simulink model "vertical_smm_with_lqr_3d"  (R2015a)
settings: Solver=FixedStepDiscrete  StartTime=0.0  StopTime=inf  FixedStep=sample_time  RelTol=1e-3
values from neighbouring files (symbols this model uses):
  forward_dx_of_dxstar = [-1.33147741515 -1.28147741462 -1.23147741409 -1.18147741356 -1.13147741303 -1.0814774125 -1.03147741197 -0.981477411445 -0.931477410916 -0.881477410388 -0.831477409975 -0.781477409737 ... (28413 elements, 41x21x33)]    [ref_trajs.mat]
  forward_x_of_dxstar = [0.245075236011 0.237749717983 0.230424199955 0.223098681927 0.215773163898 0.20844764587 0.201122127842 0.193796609813 0.186471091785 0.179145573757 0.171820055745 0.164494537786 ... (28413 elements, 41x21x33)]    [ref_trajs.mat]
  target_dx_range = [-1 -0.95 -0.9 -0.85 -0.8 -0.75 -0.7 -0.65 -0.6 -0.55 -0.5 -0.45 ... (41 elements, 1x41)]    [ref_trajs.mat]
undefined symbols (not defined in the file or in its folder): A_kalman_fourbar_gear, A_kalman_transverse, A_kalman_vertical, A_lpf_dtau, A_lpf_fourbar_angles, A_lpf_imu, A_lpf_lateral_angle, A_lpf_leg_spring, B1_lpf_dtau, B1_lpf_fourbar_angles, B1_lpf_imu, B1_lpf_lateral_angle, B1_lpf_leg_spring, B2_lpf_dtau, B2_lpf_fourbar_angles, B2_lpf_imu, B2_lpf_lateral_angle, B2_lpf_leg_spring, B_dx_versus_x0, B_kalman_fourbar_gear, B_kalman_transverse, B_kalman_vertical, backwards_K_front_of_t_row1, backwards_K_front_of_t_row2, backwards_K_sag_of_t, backwards_P_front_of_t, backwards_P_sag_of_t, C_kalman_fourbar_gear, C_kalman_transverse, C_kalman_vertical, com_leg_motor, com_torso, contact_threshold, control_start_time, d_ankle_to_foot, d_vertical_com, desired_com_forward_velocity, desired_com_lateral_velocity, desired_initial_leg_roll_left, desired_initial_leg_roll_right, desired_lateral_symmetry_angle, desired_standing_torso_pitch, desired_standing_torso_roll, desired_standing_z, desired_torso_pitch, desired_torso_roll, Discrete, fcut_contact, g, HIP_MTR_MAX_CONT_TORQUE, HIP_MTR_MAX_TORQUE, i_leg_motor, i_robot, i_torso, initial_dx_estimate, initial_dy_estimate, initial_dz_estimate, initial_z_estimate, j_motor, K_left_lat_flight ... (+72)
libraries: simulink x9, ctrlSharedLib x7
(part 1 of 5)
settings Model: CovSFcnEnable=off  Creator=wmartin  LastModifiedBy=wmartin
settings SolverCC: EnableConcurrentExecution=on
settings DataIOCC: LimitDataPoints=off  MaxDataPoints=1000000000  SaveFormat=StructureWithTime  SignalLogging=off  DSMLogging=off  VisualizeSimOutput=off
settings OptimizationCC: BlockReduction=off  OptimizeBlockIOStorage=off  BufferReuse=off  GlobalBufferReuse=off  ExpressionFolding=off  ExpressionDepthLimit=2147483647  LocalBlockOutputs=off  SimCompilerOptimization=on
settings DebuggingCC: UnderspecifiedInitializationDetection=Classic  MergeDetectMultiDrivingBlocksExec=none  SolverPrmCheckMsg=warning  StateNameClashWarn=warning
settings HardwareCC: ProdIntDivRoundTo=Zero  ProdEndianess=LittleEndian  ProdLongLongMode=on  ProdHWDeviceType=Generic->32-bit x86 compatible
settings ModelReferenceCC: UpdateModelReferenceTargets=IfOutOfDate  ModelReferenceNumInstancesAllowed=Single  ModelReferenceMinAlgLoopOccurrences=on
settings RTWCC: SystemTargetFile=slrt.tlc  TemplateMakefile=slrt_default_tmf  Description=Simulink Real-Time  RTWVerbose=off  RTWCompilerOptimization=on
settings CodeAppCC: MaxIdLength=256
settings SimulinkRealTimeCC: GeneratePreprocessorConditionals=Disable all  RL32LogBufSizeModifier=1e8

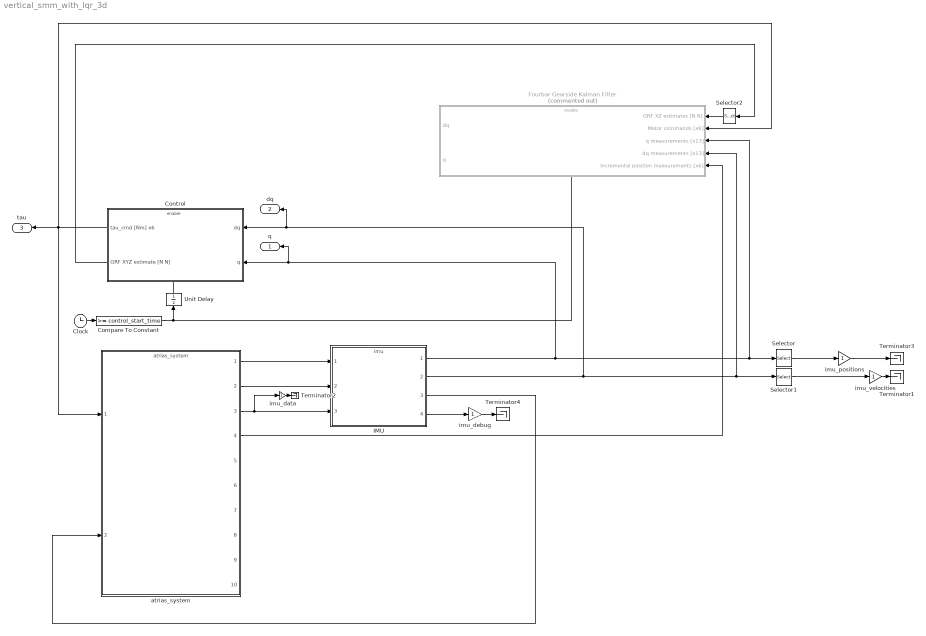
== system vertical_smm_with_lqr_3d ==
  Clock : Clock
  Compare To Constant : simulink/Logic and Bit Operations/Compare To Constant  relop=>=  const=control_start_time  OutDataTypeStr=boolean
  Control : Subsystem
  Fourbar Gearside Kalman Filter : Subsystem  Commented=on
  IMU : ModelReference  ModelNameDialog=imu  SimulationMode=Normal  ModelReferenceVersion=1.2453  CopyOfModelName=imu  DefaultDataLogging=on
  Selector : Selector  InputPortWidth=13  Indices=[11 12 13]
  Selector1 : Selector  InputPortWidth=13  Indices=[11 12 13]
  Selector2 : Selector  InputPortWidth=3  Indices=[1 3]
  Terminator{1..4} (4 alike) : Terminator
  Unit Delay : UnitDelay  SampleTime=-1
  atrias_system : ModelReference  ModelNameDialog=atrias_system  SimulationMode=Normal  ModelReferenceVersion=1.2798  CopyOfModelName=atrias_system  DefaultDataLogging=on
  imu_data : Gain
  imu_debug : Gain
  imu_positions : Gain
  imu_velocities : Gain
  q : Outport
  dq : Outport  Port=2
  tau : Outport  Port=3
  wires:
  Clock/1 -> Compare To Constant/1
  Compare To Constant/1 -> Unit Delay/1, Fourbar Gearside Kalman Filter/Enable
  imu_data/1 -> Terminator2/1
  imu_velocities/1 -> Terminator1/1
  imu_positions/1 -> Terminator3/1
  imu_debug/1 -> Terminator4/1
  IMU/4 -> imu_debug/1
  Selector/1 -> imu_positions/1
  Selector1/1 -> imu_velocities/1
  atrias_system/1 -> IMU/1
  Control/2(GRF XYZ estimate [N N]) -> Selector2/1
  IMU/1 -> q/1, Control/2(q), Fourbar Gearside Kalman Filter/3(q measurements [x13]), Selector/1
  Control/1(tau_cmd [Nm] x6) -> atrias_system/1, tau/1, Fourbar Gearside Kalman Filter/2(Motor commands [x6])
  atrias_system/2 -> IMU/2
  atrias_system/3 -> imu_data/1, IMU/3
  IMU/3 -> atrias_system/2
  Selector2/1 -> Fourbar Gearside Kalman Filter/1(GRF XZ estimates [N N])
  Unit Delay/1 -> Control/Enable
  atrias_system/4 -> Fourbar Gearside Kalman Filter/5(Incremental position measurements [x6])
  IMU/2 -> dq/1, Control/1(dq), Selector1/1, Fourbar Gearside Kalman Filter/4(dq measurements [x13])

== system vertical_smm_with_lqr_3d/Control ==
  dq : Inport
  q : Inport  Port=2
  Enable : EnablePort  StatesWhenEnabling=reset  PropagateVarSize=During execution
  Actuator Control : ModelReference  ModelNameDialog=actuator_control  SimulationMode=Normal  ModelReferenceVersion=1.160  CopyOfModelName=actuator_control  DefaultDataLogging=on
  Behavior Control : Subsystem
  Filter Velocities : Subsystem
  tau_cmd [Nm] x6 : Outport  InitialOutput=[0 0 0 0 0 0]
  GRF XYZ estimate [N N] : Outport  Port=2  InitialOutput=[0 0 0]
  wires:
  q/1 -> Actuator Control/4, Behavior Control/2(q)
  Behavior Control/1(Motor Torque Command [Nm] x6) -> Actuator Control/1
  Actuator Control/1 -> tau_cmd [Nm] x6/1
  Behavior Control/2(SEA Torque Velocity Command [Nm] x4) -> Actuator Control/2
  Behavior Control/3(Force / Position Control [1/0] x4) -> Actuator Control/3
  Behavior Control/4(GRF XYZ estimates [N N N]) -> GRF XYZ estimate [N N]/1
  Filter Velocities/1(filtered dq) -> Actuator Control/5, Behavior Control/1(dq)
  dq/1 -> Filter Velocities/1(raw dq)

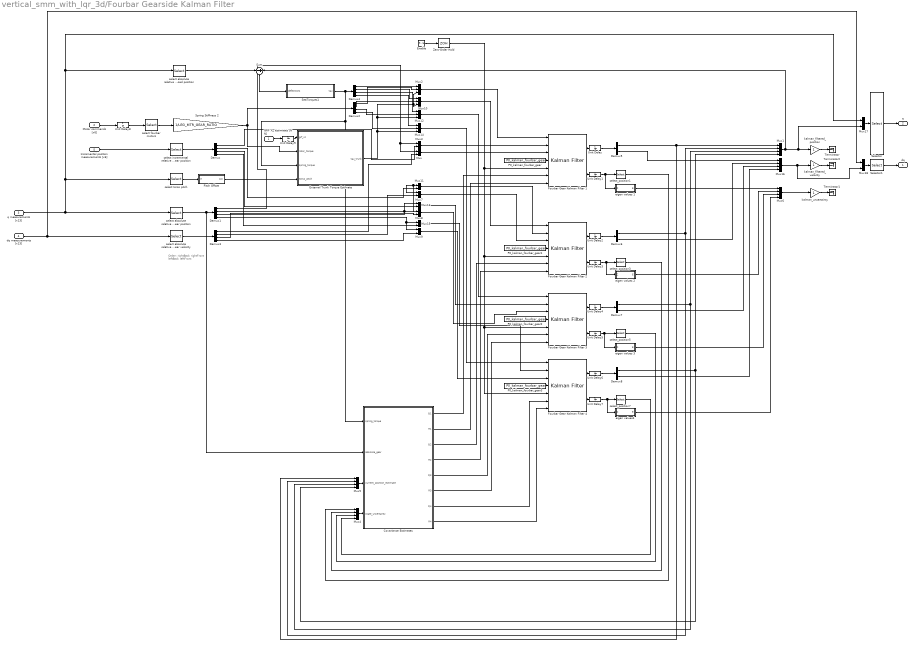
== system vertical_smm_with_lqr_3d/Fourbar Gearside Kalman Filter ==
  note: Order:
      | rightBack
      | rightFront
      | leftBack
      | leftFront
  GRF XZ estimates [N N] : Inport  SampleTime=sample_time
  Motor commands [x6] : Inport  Port=2  SampleTime=sample_time
  q measurements [x13] : Inport  Port=3  SampleTime=sample_time
  dq measurements [x13] : Inport  Port=4  SampleTime=sample_time
  Incremental position measurements [x6] : Inport  Port=5  SampleTime=sample_time
  Enable : EnablePort  ShowOutputPort=on
  Covariance Estimates : MATLAB Function  TreatAsAtomicUnit=on
  Demux{,1..4} (5 alike) : Demux
  Demux{5..8} (4 alike) : Demux  Outputs=2
  External Trunk Torque Estimate : MATLAB Function  TreatAsAtomicUnit=on
  Fourbar Gear Kalman Filter {1..4} (4 alike) : ctrlSharedLib/Kalman Filter  TimeDomain=Discrete-Time  UseCurrentEstimator=on  ModelSource=Individual A, B, C, D matrices  ModelSourceVariable=A_kf  A=A_kalman_fourbar_gear  B=B_kalman_fourbar_gear  C=C_kalman_fourbar_gear  D=0  NumberOfStates=2  NumberOfInputs=1  NumberOfOutputs=2  InitialEstimateSource=Input port  X0=initial_dx_estimate  P0=P0_kalman_transverse  UseK=off  UseGH=on  NumberOfProcessNoiseInputs=1  G=G_kalman_fourbar_gear  TimeInvariantG=on  H=0  TimeInvariantH=on  Q=1  TimeInvariantQ=off  R=1  TimeInvariantR=off  N=0  TimeInvariantN=on  AddInputPort=on  AddEnablePort=off  ExternalReset=Either  OutputEstimatedY=off  OutputP=on  Ts=sample_time
  Mux{,3,7..9,11,13,15,17..18} (10 alike) : Mux  Inputs=2
  Mux{1,4..6,16} (5 alike) : Mux
  Mux{2,10,12,14} (4 alike) : Mux  Inputs=3
  P0_kalman_fourbar_gear{,1..3} (4 alike) : Constant  Value=P0_kalman_fourbar_gear
  Pitch Offset : Subsystem
  SeaTorques1 : MATLAB Function  TreatAsAtomicUnit=on
  Selector : Selector  InputPortWidth=17  Indices=[1 14 3 15 5 16 7 17 9 10 11 12 13]
  Selector1 : Selector  InputPortWidth=17  Indices=[1 14 3 15 5 16 7 17 9 10 11 12 13]
  Spring Stiffness 2 : Gain  Gain=1/LEG_MTR_GEAR_RATIO
  Sum : Sum  Inputs=-|+
  Terminator : Terminator
  Terminator1 : Terminator
  Terminator2 : Terminator
  Unit Delay{,1..9} (10 alike) : UnitDelay  SampleTime=-1
  Zero-Order Hold : ZeroOrderHold  SampleTime=sample_time
  eigen values 1 : MATLAB Function  TreatAsAtomicUnit=on
  eigen values 2 : MATLAB Function  TreatAsAtomicUnit=on
  eigen values 3 : MATLAB Function  TreatAsAtomicUnit=on
  "eigen values4 " : MATLAB Function  TreatAsAtomicUnit=on
  kalman_filtered_position : Gain
  kalman_filtered_velocity : Gain
  kalman_uncertainty : Gain
  select absolute relative gear position : Selector  InputPortWidth=13  Indices=[2 4 6 8]
  select absolute relative gear velocity : Selector  InputPortWidth=13  Indices=[2 4 6 8]
  select absolute relative load position : Selector  InputPortWidth=13  Indices=[2 4 6 8]
  select fourbar motors : Selector  InputPortWidth=6  Indices=[1 2 3 4]
  select incremental relative gear position : Selector  InputPortWidth=6  Indices=[1 2 3 4]
  select torso pitch : Selector  InputPortWidth=13  Indices=[13]
  select_position{1,3,5,7} (4 alike) : Selector  NumberOfDimensions=2  InputPortWidth=2  IndexOptions=Index vector (dialog),Index vector (dialog)  Indices=[1],[1]  OutputSizes=1,1
  dq : Outport
  q : Outport  Port=2
  wires:
  select incremental relative gear position/1 -> Demux/1
  q measurements [x13]/1 -> select absolute relative gear position/1, Mux17/1, select absolute relative load position/1, select torso pitch/1
  Incremental position measurements [x6]/1 -> select incremental relative gear position/1
  Motor commands [x6]/1 -> Unit Delay8/1
  select fourbar motors/1 -> Spring Stiffness 2/1
  P0_kalman_fourbar_gear/1 -> Fourbar Gear Kalman Filter 1/4
  Mux/1 -> Fourbar Gear Kalman Filter 1/3
  select absolute relative gear velocity/1 -> Demux3/1
  dq measurements [x13]/1 -> Mux18/1, select absolute relative gear velocity/1
  Demux3/1 -> Mux/2
  GRF XZ estimates [N N]/1 -> Unit Delay9/1
  SeaTorques1/1(tau) -> Demux4/1, External Trunk Torque Estimate/3(spring_torque), Covariance Estimates/1(spring_torque)
  Fourbar Gear Kalman Filter 1/1 -> Unit Delay/1
  Demux5/1 -> Mux1/1, Mux5/1
  Mux1/1 -> Sum/2, Mux17/2, kalman_filtered_position/1
  select absolute relative load position/1 -> Sum/1
  Sum/1 -> SeaTorques1/1(deflections)
  External Trunk Torque Estimate/1(tau_trunk) -> Mux2/3, Mux10/3, Mux12/3, Mux14/3
  Demux4/1 -> Mux2/1
  Demux2/1 -> Mux2/2
  Mux2/1 -> Fourbar Gear Kalman Filter 1/1
  Demux/1 -> Mux3/2
  Demux1/1 -> Mux3/1, Mux/1
  Mux3/1 -> Fourbar Gear Kalman Filter 1/2
  Fourbar Gear Kalman Filter 1/2 -> Unit Delay1/1
  Mux4/1 -> Covariance Estimates/4(state_uncertainty)
  select absolute relative gear position/1 -> Covariance Estimates/2(absolute_gear), Demux1/1
  Mux5/1 -> Covariance Estimates/3(current_position_estimate)
  Covariance Estimates/1(Q1) -> Fourbar Gear Kalman Filter 1/6
  Covariance Estimates/2(R1) -> Fourbar Gear Kalman Filter 1/7
  select torso pitch/1 -> Pitch Offset/1(in)
  select_position1/1 -> Mux4/1
  P0_kalman_fourbar_gear1/1 -> Fourbar Gear Kalman Filter 2/4
  Fourbar Gear Kalman Filter 2/1 -> Unit Delay2/1
  Fourbar Gear Kalman Filter 2/2 -> Unit Delay3/1
  P0_kalman_fourbar_gear2/1 -> Fourbar Gear Kalman Filter 3/4
  Fourbar Gear Kalman Filter 3/1 -> Unit Delay4/1
  Fourbar Gear Kalman Filter 3/2 -> Unit Delay5/1
  P0_kalman_fourbar_gear3/1 -> Fourbar Gear Kalman Filter 4/4
  Fourbar Gear Kalman Filter 4/1 -> Unit Delay6/1
  Fourbar Gear Kalman Filter 4/2 -> Unit Delay7/1
  Covariance Estimates/3(Q2) -> Fourbar Gear Kalman Filter 2/6
  Covariance Estimates/5(Q3) -> Fourbar Gear Kalman Filter 3/6
  Covariance Estimates/7(Q4) -> Fourbar Gear Kalman Filter 4/6
  Covariance Estimates/4(R2) -> Fourbar Gear Kalman Filter 2/7
  Covariance Estimates/6(R3) -> Fourbar Gear Kalman Filter 3/7
  Covariance Estimates/8(R4) -> Fourbar Gear Kalman Filter 4/7
  select_position3/1 -> Mux4/2
  select_position5/1 -> Mux4/3
  select_position7/1 -> Mux4/4
  Demux6/1 -> Mux5/2, Mux1/2
  Demux7/1 -> Mux1/3, Mux5/3
  Demux8/1 -> Mux1/4, Mux5/4
  kalman_filtered_position/1 -> Terminator/1
  Enable/1 -> Zero-Order Hold/1
  Mux7/1 -> Fourbar Gear Kalman Filter 2/3
  Mux8/1 -> Fourbar Gear Kalman Filter 3/3
  Mux9/1 -> Fourbar Gear Kalman Filter 4/3
  Mux10/1 -> Fourbar Gear Kalman Filter 2/1
  Mux11/1 -> Fourbar Gear Kalman Filter 2/2
  Mux13/1 -> Fourbar Gear Kalman Filter 3/2
  Mux12/1 -> Fourbar Gear Kalman Filter 3/1
  Mux15/1 -> Fourbar Gear Kalman Filter 4/2
  Mux14/1 -> Fourbar Gear Kalman Filter 4/1
  Demux3/2 -> Mux7/2
  Demux3/3 -> Mux8/2
  Demux3/4 -> Mux9/2
  Demux1/2 -> Mux7/1, Mux11/1
  Demux1/3 -> Mux13/1, Mux8/1
  Demux1/4 -> Mux9/1, Mux15/1
  Demux/2 -> Mux11/2
  Demux/3 -> Mux13/2
  Demux/4 -> Mux15/2
  Demux4/2 -> Mux10/1
  Demux4/3 -> Mux12/1
  Demux4/4 -> Mux14/1
  Demux2/2 -> Mux10/2
  Demux2/3 -> Mux12/2
  Demux2/4 -> Mux14/2
  kalman_uncertainty/1 -> Terminator1/1
  Mux6/1 -> kalman_uncertainty/1
  kalman_filtered_velocity/1 -> Terminator2/1
  Mux16/1 -> Mux18/2, kalman_filtered_velocity/1
  Demux5/2 -> Mux16/1
  Demux6/2 -> Mux16/2
  Demux7/2 -> Mux16/3
  Demux8/2 -> Mux16/4
  Zero-Order Hold/1 -> Fourbar Gear Kalman Filter 4/5, Fourbar Gear Kalman Filter 3/5, Fourbar Gear Kalman Filter 2/5, Fourbar Gear Kalman Filter 1/5
  Unit Delay1/1 -> eigen values 1/1(Z), select_position1/1
  Unit Delay3/1 -> eigen values 2/1(Z), select_position3/1
  Unit Delay4/1 -> Demux7/1
  Unit Delay7/1 -> "eigen values4 "/1(Z), select_position7/1
  Unit Delay6/1 -> Demux8/1
  Spring Stiffness 2/1 -> Demux2/1, External Trunk Torque Estimate/2(rotor_torque)
  Unit Delay5/1 -> eigen values 3/1(Z), select_position5/1
  eigen values 1/1(E) -> Mux6/1
  eigen values 2/1(E) -> Mux6/2
  eigen values 3/1(E) -> Mux6/3
  "eigen values4 "/1(E) -> Mux6/4
  Unit Delay/1 -> Demux5/1
  Unit Delay2/1 -> Demux6/1
  Mux17/1 -> Selector/1
  Selector/1 -> q/1
  Selector1/1 -> dq/1
  Mux18/1 -> Selector1/1
  Unit Delay8/1 -> select fourbar motors/1
  Unit Delay9/1 -> External Trunk Torque Estimate/1(grf_xz)
  Pitch Offset/1(out) -> External Trunk Torque Estimate/4(torso_pitch)

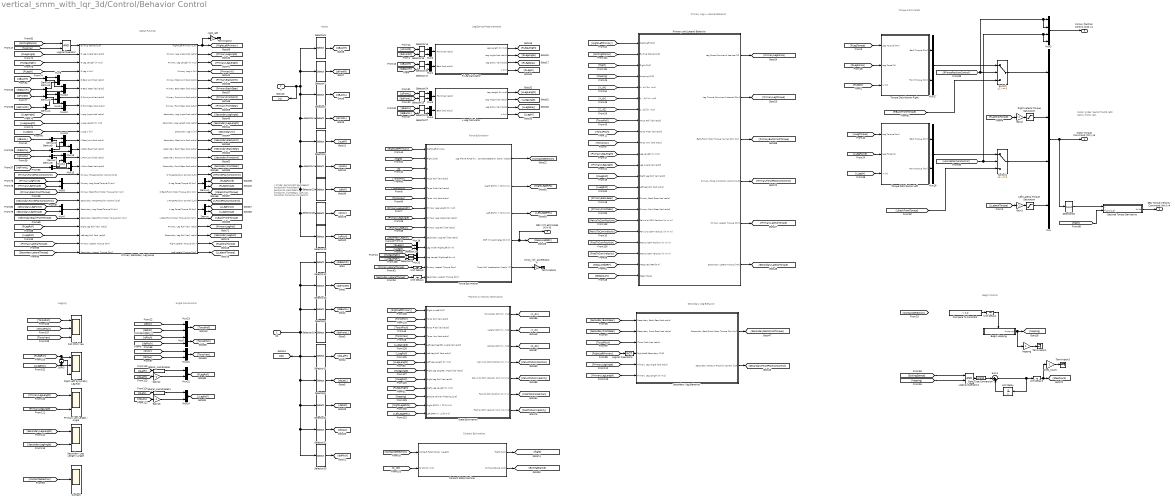
== system vertical_smm_with_lqr_3d/Control/Behavior Control ==
  note: Signal Routing
  note: Begin Control
  note: Position & Velocity Estimation
  note: Force Estimation
  note: Leg/Spring Measurements
  note: Torque Commands
  note: Secondary Leg Behavior
  note: Primary Leg + Lateral Behavior
  note: Inputs
  note: q Order:
      |
      | backJointR
      | backGearR
      | frontJointR
      | frontGearR
      |
      | backJointL
      | backGearL
      | frontJointL
      | frontGearL
      |
      | latR
      | latL
      |
      | torsoRoll
      | torsoYaw
      | torsoPitch
  note: Motor Order:
      |
      | backR
      | frontR
      | latR
      | backL
      | frontL
      | latL
  note: Angle Conversions
  note: Contact Estimation
  note: Logging
  dq : Inport
  q : Inport  Port=2
  Begin Hopping : Subsystem
  Compare To Constant : simulink/Logic and Bit Operations/Compare To Constant  relop=>  const=1.2  OutDataTypeStr=boolean
  Contact : Scope
      settings: YMin=0.3  YMax=0.9  SaveName=ScopeData11  SampleInput=on
  Contact State Machine : Subsystem
  Data Type Conversion : DataTypeConversion  OutDataTypeStr=uint32
  Demux{,1,3..10} (10 alike) : Demux  Outputs=2
  Desired Torque Derivative : Subsystem
  Force Estimation : Subsystem
  Gain{1..2,12..13} (4 alike) : Gain  Gain=-1
  L Leg Calculator : Subsystem
  Left Lateral Torque Saturation : Saturate  UpperLimit=max_torque_lateral  LowerLimit=-max_torque_lateral
      settings: AttributesFormatString=Top: %<UpperLimit>\nBottom: %<LowerLimit>
  Logical Operator : Logic  IconShape=distinctive  AllPortsSameDT=off  OutDataTypeStr=boolean
  Logical Operator1 : Logic  AllPortsSameDT=off  OutDataTypeStr=boolean
  Logical Operator3 : Logic  Operator=NOT  AllPortsSameDT=off  OutDataTypeStr=boolean
  Mux : Mux
  Mux{1..2,4..24} (23 alike) : Mux  Inputs=2
  Mux3 : Mux
  Primary Leg Length / Angle : Scope  NumInputPorts=2
      settings: YMin=0.3~0  YMax=0.9~3.5  SaveName=ScopeData21  SampleInput=on
  Primary Secondary Leg Swap : Subsystem
  Primary and Lateral Behavior : Subsystem
  R Leg Calculator : Subsystem
  Right Lateral Torque Saturation : Saturate  UpperLimit=max_torque_lateral  LowerLimit=-max_torque_lateral
      settings: AttributesFormatString=Top: %<UpperLimit>\nBottom: %<LowerLimit>
  Right Left Symmetry Leg Roll : Scope  NumInputPorts=3
      settings: YMin=-0.2~-0.5~-0.5  YMax=1.3~1.8~0.5  SaveName=ScopeData19  SampleInput=on
  Roll Pitch Yaw : Scope  NumInputPorts=3
      settings: YMin=-1000~-5~-5  YMax=1000~5~5  SampleInput=on
  Secondary Leg Behavior : Subsystem
  Secondary Leg Length / Angle : Scope  NumInputPorts=2
      settings: YMin=-1~-0.8  YMax=1~1.4  SaveName=ScopeData22  SampleInput=on
  Selector1 : Selector  InputPortWidth=13  Indices=[10]
  Selector10 : Selector  InputPortWidth=13  Indices=[7 8]
  Selector11 : Selector  InputPortWidth=13  Indices=[9]
  Selector12 : Selector  InputPortWidth=13  Indices=[1 2]
  Selector13 : Selector  InputPortWidth=13  Indices=[3 4]
  Selector{14..17,19,24..27,29} (10 alike) : Selector  InputPortWidth=2  Indices=[1]
  Selector18 : Selector  InputPortWidth=13  Indices=[13]
  Selector2 : Selector  InputPortWidth=13  Indices=[5 6]
  Selector20 : Selector  InputPortWidth=13  Indices=[13]
  Selector21 : Selector  InputPortWidth=13  Indices=[11]
  Selector22 : Selector  InputPortWidth=13  Indices=[12]
  Selector23 : Selector  InputPortWidth=13  Indices=[11]
  Selector28 : Selector  InputPortWidth=13  Indices=[12]
  Selector33 : Selector  InputPortWidth=6  Indices=[1 2 4 5]
  Selector4 : Selector  InputPortWidth=13  Indices=[7 8]
  Selector5 : Selector  InputPortWidth=13  Indices=[9]
  Selector6 : Selector  InputPortWidth=13  Indices=[1 2]
  Selector7 : Selector  InputPortWidth=13  Indices=[3 4]
  Selector8 : Selector  InputPortWidth=13  Indices=[10]
  Selector9 : Selector  InputPortWidth=13  Indices=[5 6]
  State Estimation : Subsystem
  Sum1 : Sum  Inputs=|++  OutMin=0
  Sum3 : Sum  Inputs=-|+
  Switch : Switch  Criteria=u2 ~= 0
  Switch1 : Switch  Criteria=u2 ~= 0
  Terminator{1..3,6} (4 alike) : Terminator
  Torque Distribution Left : Subsystem
  Torque Distribution Right : Subsystem
  Unit Delay : UnitDelay  SampleTime=-1
  Unit Delay{1..4} (4 alike) : UnitDelay  SampleTime=sample_time
  hopping : Gain
  lateral_coordinates : Fcn  Expr=pi/2-u
  lateral_coordinates1 : Fcn  Expr=pi/2-u
  right_left : Gain
  step_count : Gain
  torso_roll_acceleration : Gain
  Motor Torque Command [Nm] x6 : Outport  OutputWhenDisabled=reset  InitialOutput=[0 0 0 0 0 0]
  SEA Torque Velocity Command [Nm] x4 : Outport  Port=2  OutputWhenDisabled=reset  InitialOutput=[0 0 0 0 0 0]
  Force / Position Control [1/0] x4 : Outport  Port=3  OutputWhenDisabled=reset  InitialOutput=[0 0 0 0 0 0]
  GRF XYZ estimates [N N N] : Outport  Port=4  OutputWhenDisabled=reset  InitialOutput=[0 0 0 0 0 0]
  wires:
  Unit Delay1/1 -> Begin Hopping/Enable
  Data Type Conversion/1 -> Sum1/1
  Logical Operator1/1 -> Data Type Conversion/1
  Sum1/1 -> Unit Delay/1, Unit Delay2/1
  Unit Delay/1 -> Sum1/2
  Switch1/1 -> Mux/3
  [LBackFrontTorque] -> Switch1/3
  Mux18/1 -> Switch1/1
  [RBackFrontTorque] -> Switch/3
  Mux17/1 -> Switch/1
  Torque Distribution Left/2(Front Torque [Nm]) -> Mux18/2
  Torque Distribution Left/1(Back Torque [Nm]) -> Mux18/1
  Torque Distribution Right/1(Back Torque [Nm]) -> Mux17/1
  Torque Distribution Right/2(Front Torque [Nm]) -> Mux17/2
  [RLateralTorque] -> Gain2/1
  Switch/1 -> Mux/1
  [LForcePositionControl] -> Switch1/2, Mux3/3, Mux3/4
  [RForcePositionControl] -> Switch/2, Mux3/1, Mux3/2
  [SecondaryBackGear] -> Secondary Leg Behavior/1(Secondary Back Gear [rad rad/s])
  [SecondaryFrontGear] -> Secondary Leg Behavior/2(Secondary Front Gear [rad rad/s])
  Logical Operator3/1 -> Secondary Leg Behavior/4(Right/Left Secondary [1/0])
  [RightLeftPrimary] -> Logical Operator3/1
  Primary and Lateral Behavior/4(Primary Force or Position Control [1/0]) -> [PrimaryForcePositionControl]
  Primary and Lateral Behavior/3(Back/Front Motor Torque (swing) [Nm Nm]) -> [PrimaryBackFrontTorque]
  Primary Secondary Leg Swap/1(Right/Left Primary [1/0]) -> right_left/1, [RightLeftPrimary]
  Logical Operator/1 -> Primary Secondary Leg Swap/1(Exiting Stance [1/0])
  Primary Secondary Leg Swap/21(L Back/Front Motor Torque [Nm Nm]) -> [LBackFrontTorque]
  Primary Secondary Leg Swap/18(R Back/Front Motor Torque [Nm Nm]) -> [RBackFrontTorque]
  Primary Secondary Leg Swap/16(R Force/Position Control [1/0]) -> [RForcePositionControl]
  Primary Secondary Leg Swap/19(L Force/Position Control [1/0]) -> [LForcePositionControl]
  Primary Secondary Leg Swap/11(Secondary Leg w [m]) -> [SecondaryW]
  Primary Secondary Leg Swap/15(Secondary Front Gear [rad rad/s]) -> [SecondaryFrontGear]
  Primary Secondary Leg Swap/14(Secondary Front Joint [rad rad/s]) -> [SecondaryFrontJoint]
  Primary Secondary Leg Swap/13(Secondary Back Gear [rad rad/s]) -> [SecondaryBackGear]
  Primary Secondary Leg Swap/12(Secondary Back Joint [rad rad/s]) -> [SecondaryBackJoint]
  Primary Secondary Leg Swap/8(Primary Front Gear [rad rad/s]) -> [PrimaryFrontGear]
  Primary Secondary Leg Swap/7(Primary Front Joint [rad rad/s]) -> [PrimaryFrontJoint]
  Primary Secondary Leg Swap/6(Primary Back Gear [rad rad/s]) -> [PrimaryBackGear]
  Primary Secondary Leg Swap/5(Primary Back Joint [rad rad/s]) -> [PrimaryBackJoint]
  [SecondaryBackFrontTorque] -> Primary Secondary Leg Swap/21(Secondary Back/Front Motor Torque [Nm Nm])
  [PrimaryBackFrontTorque] -> Primary Secondary Leg Swap/18(Primary Back/Front Motor Torque [Nm Nm])
  [SecondaryForcePositionControl] -> Primary Secondary Leg Swap/19(Secondary Force/Position Control [1/0])
  [PrimaryForcePositionControl] -> Primary Secondary Leg Swap/16(Primary Force/Position Control [1/0])
  Demux9/2 -> Mux13/2
  Demux9/1 -> Mux16/2
  Demux10/2 -> Mux13/1
  Demux10/1 -> Mux16/1
  [qBackL] -> Demux10/1
  [dqBackL] -> Demux9/1
  Demux8/2 -> Mux15/2
  Demux8/1 -> Mux14/2
  Demux7/2 -> Mux15/1
  Demux7/1 -> Mux14/1
  Mux15/1 -> Primary Secondary Leg Swap/15(L Front Gear [rad rad/s])
  Mux14/1 -> Primary Secondary Leg Swap/14(L Front Joint [rad rad/s])
  Mux13/1 -> Primary Secondary Leg Swap/13(L Back Gear [rad rad/s])
  Mux16/1 -> Primary Secondary Leg Swap/12(L Back Joint [rad rad/s])
  [dqFrontL] -> Demux8/1
  [qFrontL] -> Demux7/1
  Demux5/2 -> Mux10/2
  Demux5/1 -> Mux9/2
  Demux6/2 -> Mux10/1
  Demux6/1 -> Mux9/1
  [qBackR] -> Demux6/1
  [dqBackR] -> Demux5/1
  Demux4/2 -> Mux12/2
  Demux4/1 -> Mux11/2
  Demux3/2 -> Mux12/1
  Demux3/1 -> Mux11/1
  Mux12/1 -> Primary Secondary Leg Swap/8(R Front Gear [rad rad/s])
  Mux11/1 -> Primary Secondary Leg Swap/7(R Front Joint [rad rad/s])
  Mux10/1 -> Primary Secondary Leg Swap/6(R Back Gear [rad rad/s])
  Mux9/1 -> Primary Secondary Leg Swap/5(R Back Joint [rad rad/s])
  [dqFrontR] -> Demux4/1
  [qFrontR] -> Demux3/1
  Demux1/2 -> [RLegTorque]
  Demux1/1 -> [RLegForce]
  Primary Secondary Leg Swap/17(R Leg Force/Torque [N Nm]) -> Demux1/1
  Demux/2 -> [LLegTorque]
  Demux/1 -> [LLegForce]
  Primary Secondary Leg Swap/20(L Leg Force/Torque [N Nm]) -> Demux/1
  Primary Secondary Leg Swap/9(Secondary Leg Angle [rad rad/s]) -> [SecondaryLegAngle]
  Primary Secondary Leg Swap/10(Secondary Leg Length [rad rad/s]) -> [SecondaryLegLength]
  [PrimaryLegForce] -> Mux8/1
  [PrimaryLegTorque] -> Mux8/2
  Mux8/1 -> Primary Secondary Leg Swap/17(Primary Leg Force/Torque [N Nm])
  Mux6/1 -> Primary Secondary Leg Swap/20(Secondary Leg Force/Torque [N Nm])
  [SecondaryLegTorque] -> Mux6/2
  [SecondaryLegForce] -> Mux6/1
  [LLegW] -> Primary Secondary Leg Swap/11(L Leg w [m])
  [LLegLength] -> Primary Secondary Leg Swap/10(L Leg Length [m m/s])
  [LLegAngle] -> Primary Secondary Leg Swap/9(L Leg Angle [rad rad/s])
  [RLegW] -> Primary Secondary Leg Swap/4(R Leg w [m])
  [RLegLength] -> Primary Secondary Leg Swap/3(R Leg Length [m m/s])
  [RLegAngle] -> Primary Secondary Leg Swap/2(R Leg Angle [rad rad/s])
  Primary Secondary Leg Swap/3(Primary Leg Length [m m/s]) -> [PrimaryLegLength]
  Primary Secondary Leg Swap/4(Primary Leg w [m]) -> [PrimaryW]
  Primary Secondary Leg Swap/2(Primary Leg Angle [rad rad/s]) -> [PrimaryLegAngle]
  Mux3/1 -> Force / Position Control [1/0] x4/1
  [TorsoPitch] -> Secondary Leg Behavior/3(Torso Pitch [rad rad/s])
  Compare To Constant/1 -> Unit Delay1/1
  right_left/1 -> Terminator2/1
  [LLegW] -> Torque Distribution Left/3(w [m])
  [LLegTorque] -> Torque Distribution Left/1(Leg Torque [Nm])
  hopping/1 -> Terminator1/1
  Primary and Lateral Behavior/2(Leg Torque Command (stance) [Nm]) -> [PrimaryLegTorque]
  Primary and Lateral Behavior/1(Leg Force Command (stance) [N]) -> [PrimaryLegForce]
  L Leg Calculator/4(w [m]) -> [LLegW]
  R Leg Calculator/4(w [m]) -> [RLegW]
  Selector26/1 -> Mux4/1
  Selector27/1 -> Mux4/2
  Selector25/1 -> Mux5/2
  Selector24/1 -> Mux5/1
  L Leg Calculator/3(Leg Splay [rad rad/s]) -> [LLegSplay]
  L Leg Calculator/2(Leg Angle [rad rad/s]) -> [LLegAngle]
  L Leg Calculator/1("Leg Length [m m/s] ") -> [LLegLength]
  Mux4/1 -> L Leg Calculator/2(Back [rad rad/s])
  Mux5/1 -> L Leg Calculator/1(Front [rad rad/s])
  [dqFrontL] -> Selector25/1
  [qFrontL] -> Selector24/1
  [dqBackL] -> Selector27/1
  [qBackL] -> Selector26/1
  Selector23/1 -> [qRoll]
  [RLegTorque] -> Torque Distribution Right/1(Leg Torque [Nm])
  Selector18/1 -> [qPitch]
  q/1 -> [q], Selector1/1, Selector23/1, Selector28/1, Selector18/1, Selector5/1, Selector4/1, Selector2/1, Selector7/1, Selector6/1
  Selector16/1 -> Mux1/1
  Selector17/1 -> Mux1/2
  Selector15/1 -> Mux2/2
  Selector14/1 -> Mux2/1
  [RLegW] -> Torque Distribution Right/3(w [m])
  R Leg Calculator/3(Leg Splay [rad rad/s]) -> [RLegSplay]
  R Leg Calculator/2(Leg Angle [rad rad/s]) -> [RLegAngle]
  R Leg Calculator/1("Leg Length [m m/s] ") -> [RLegLength]
  Mux1/1 -> R Leg Calculator/2(Back [rad rad/s])
  Mux2/1 -> R Leg Calculator/1(Front [rad rad/s])
  [dqFrontR] -> Selector15/1
  [qFrontR] -> Selector14/1
  [dqBackR] -> Selector17/1
  [qBackR] -> Selector16/1
  Selector5/1 -> [qLatR]
  Selector1/1 -> [qLatL]
  Selector6/1 -> [qBackR]
  Selector7/1 -> [qFrontR]
  Selector2/1 -> [qBackL]
  Selector4/1 -> [qFrontL]
  [PrimaryLegAngle] -> Secondary Leg Behavior/5(Primary Leg Angle [rad rad/s])
  Selector33/1 -> Desired Torque Derivative/1(x)
  Desired Torque Derivative/1(dx/dt) -> SEA Torque Velocity Command [Nm] x4/1
  Mux/1 -> Selector33/1, Motor Torque Command [Nm] x6/1
  [PrimaryLegLength] -> Secondary Leg Behavior/6(Primary Leg Length [m m/s])
  Selector28/1 -> [qYaw]
  Force Estimation/1(Leg Plane Force for Contact Detection [body weight]) -> [ContactDetection]
  State Estimation/1("Horizontal COM [m, m/s]") -> [X_dX]
  State Estimation/3("Vertical COM [m, m/s]") -> [Z_dZ]
  [RLegLength] -> State Estimation/10(Right Leg Length [m m/s])
  [TorsoRoll] -> State Estimation/2(Torso Roll [rad rad/s])
  [TorsoPitch] -> State Estimation/3(Torso Pitch [rad rad/s])
  [RLegRoll] -> State Estimation/9(Right Leg Roll [rad rad/s])
  [LLegRoll] -> State Estimation/6(Left Leg Roll [rad rad/s])
  [LLegLength] -> State Estimation/7(Left Leg Length [m m/s])
  [LLegAngle] -> State Estimation/5(Left Leg Sagittal Angle [rad rad/s])
  [RLegAngle] -> State Estimation/8(Right Leg Sagittal Angle [rad rad/s])
  [RightLeftPrimary] -> State Estimation/1(Right or Left [1/0])
  [hopping] -> State Estimation/11(Enable Kalman Filtering [1/0])
  Force Estimation/2(Right GRF [X Y Z] [N N N]) -> [RightLegGRFs]
  [RightLegGRFs] -> State Estimation/12(Right GRF [X Y Z] [N N N])
  [LeftLegGRFs] -> State Estimation/13(Left GRF [X Y Z] [N N N])
  [LLateralTorque] -> Gain1/1
  Force Estimation/3(Left GRF [X Y Z] [N N N]) -> [LeftLegGRFs]
  [LLegForce] -> Torque Distribution Left/2(Leg Force [N])
  [RLegForce] -> Torque Distribution Right/2(Leg Force [N])
  Force Estimation/4(GRF XYZ estimates [N N N]) -> GRF XYZ estimates [N N N]/1, [MeasuredGRF]
  Primary Secondary Leg Swap/22("Primary Leg Roll [rad, rad/s]") -> [PrimaryLegRoll]
  Primary Secondary Leg Swap/23("Secondary Leg Roll [rad, rad/s]") -> [SecondaryLegRoll]
  [RLegRoll] -> Primary Secondary Leg Swap/22("Right Leg Roll [rad, rad/s]")
  [LLegRoll] -> Primary Secondary Leg Swap/23("Left Leg Roll [rad, rad/s]")
  State Estimation/4(Pelvis to COM Position [m m m]) -> [PelvisToComPosition]
  State Estimation/5(Pelvis to COM Velocity [m/s m/s m/s]) -> [PelvisToComVelocity]
  step_count/1 -> Terminator3/1
  Unit Delay2/1 -> step_count/1, [StepCount]
  State Estimation/2("Lateral COM [m, m/s]") -> [Y_dY]
  [ExitingStance] -> Logical Operator1/1
  [hopping] -> Logical Operator1/2
  [hopping] -> Logical Operator/2
  [ExitingStance] -> Logical Operator/1
  [TorsoYaw] -> State Estimation/4(Torso Yaw [rad rad/s])
  [RightLeftPrimary] -> Force Estimation/1(Right/Left Primary)
  [flight] -> Force Estimation/2(Flight [1/0])
  [TorsoRoll] -> Force Estimation/4(Torso Roll [rad rad/s])
  [TorsoYaw] -> Force Estimation/6(Torso Yaw [rad rad/s])
  [TorsoPitch] -> Force Estimation/5(Torso Pitch [rad rad/s])
  [q] -> Force Estimation/3(q)
  [PrimaryLegLength] -> Force Estimation/7(Primary Leg Length [m m/s])
  [PrimaryLegAngle] -> Force Estimation/8(Primary Leg Angle [rad rad/s])
  [PrimaryLegRoll] -> Force Estimation/9(Primary Leg Roll [rad rad/s])
  [RLegW] -> Mux19/1
  [LLegW] -> Mux19/2
  Mux19/1 -> Force Estimation/11(Leg Width Right/Left [m m])
  [RLegLength] -> Selector19/1
  Mux20/1 -> Force Estimation/12(Leg Length Right/Left [m m])
  [SecondaryLegRoll] -> Force Estimation/10(Secondary Leg Roll [rad rad/s])
  [PrimaryLateralTorque] -> Unit Delay3/1
  [SecondaryLateralTorque] -> Unit Delay4/1
  torso_roll_acceleration/1 -> Terminator6/1
  Force Estimation/5(Torso Roll Acceleration [rad/s^2]) -> torso_roll_acceleration/1
  [PrimaryLateralTorque] -> Primary Secondary Leg Swap/24(Primary Lateral Torque [Nm])
  [SecondaryLateralTorque] -> Primary Secondary Leg Swap/25(Secondary Lateral Torque [Nm])
  Primary Secondary Leg Swap/24(Right Lateral Torque [Nm]) -> [RLateralTorque]
  Primary Secondary Leg Swap/25(Left Lateral Torque [Nm]) -> [LLateralTorque]
  Right Lateral Torque Saturation/1 -> Mux/2
  Left Lateral Torque Saturation/1 -> Mux/4
  Primary and Lateral Behavior/6(Secondary Lateral Torque [Nm]) -> [SecondaryLateralTorque]
  Primary and Lateral Behavior/5(Primary Lateral Torque [Nm]) -> [PrimaryLateralTorque]
  Selector19/1 -> Mux20/1
  [LLegLength] -> Selector29/1
  Selector29/1 -> Mux20/2
  Unit Delay3/1 -> Force Estimation/13(Primary Lateral Torque [Nm])
  Unit Delay4/1 -> Force Estimation/14(Secondary Lateral Torque [Nm])
  Begin Hopping/1(Hopping?) -> [hopping], hopping/1
  Gain2/1 -> Right Lateral Torque Saturation/1
  Gain1/1 -> Left Lateral Torque Saturation/1
  [flight] -> Desired Torque Derivative/2(flight [1/0])
  State Estimation/6(Foot to COM Position [m m m]) -> [FootToComPosition]
  State Estimation/7(Foot to COM Velocity [m/s m/s m/s]) -> [FootToComVelocity]
  [TorsoYaw] -> Primary and Lateral Behavior/10(Torso Yaw [rad rad/s])
  [LLegRoll] -> Primary and Lateral Behavior/14(Left Leg Roll [rad rad/s])
  [RLegRoll] -> Primary and Lateral Behavior/13(Right Leg Roll [rad rad/s])
  [Y_dY] -> Primary and Lateral Behavior/6("[y,  dy] [m, m/s]")
  [StepCount] -> Primary and Lateral Behavior/22(Steps Taken)
  [MeasuredGRF] -> Primary and Lateral Behavior/21(Measured GRF [N N])
  [TorsoRoll] -> Primary and Lateral Behavior/8(Torso Roll [rad rad/s])
  [Z_dZ] -> Primary and Lateral Behavior/7("[z, dz] [m, m/s]")
  [X_dX] -> Primary and Lateral Behavior/5("[x, dx] [m, m/s]")
  [PelvisToComVelocity] -> Primary and Lateral Behavior/18(Pelvis to COM Velocity [m m m])
  [PelvisToComPosition] -> Primary and Lateral Behavior/17(Pelvis to COM Position [m m m])
  [TorsoPitch] -> Primary and Lateral Behavior/9(Torso Pitch [rad rad/s])
  [PrimaryFrontGear] -> Primary and Lateral Behavior/16(Primary Front Gear [rad rad/s])
  [PrimaryLegLength] -> Primary and Lateral Behavior/11(Leg Length [m m/s])
  [hopping] -> Primary and Lateral Behavior/4(Hopping [1/0])
  [RightLeftPrimary] -> Primary and Lateral Behavior/1(Right/Left [1/0])
  [PrimaryBackGear] -> Primary and Lateral Behavior/15(Primary Back Gear [rad rad/s])
  [PrimaryLegAngle] -> Primary and Lateral Behavior/12(Leg Angle [rad rad/s])
  Contact State Machine/1(flight [1/0]) -> [flight]
  [FootToComVelocity] -> Primary and Lateral Behavior/20(Foot to COM Velocity [m m m])
  [FootToComPosition] -> Primary and Lateral Behavior/19(Foot to COM Position [m m m])
  Contact State Machine/2(Exiting Stance [1/0]) -> [ExitingStance]
  [flight] -> Primary and Lateral Behavior/3(Flight [1/0])
  [ContactDetection] -> Contact State Machine/1(Contact Factor [body weight])
  [Z_dZ] -> Contact State Machine/2("[Z dZ] [m m/s]")
  [ExitingStance] -> Primary and Lateral Behavior/2(Exiting Stance [1/0])
  [TorsoYaw] -> Roll Pitch Yaw/3
  [TorsoPitch] -> Roll Pitch Yaw/2
  [TorsoRoll] -> Roll Pitch Yaw/1
  [LLegRoll] -> Sum3/2, Right Left Symmetry Leg Roll/2
  [RLegRoll] -> Sum3/1, Right Left Symmetry Leg Roll/1
  Sum3/1 -> Right Left Symmetry Leg Roll/3
  [PrimaryLegLength] -> Primary Leg Length / Angle/1
  [PrimaryLegAngle] -> Primary Leg Length / Angle/2
  [SecondaryLegLength] -> Secondary Leg Length / Angle/1
  [SecondaryLegAngle] -> Secondary Leg Length / Angle/2
  [ContactDetection] -> Contact/1
  Secondary Leg Behavior/1(Secondary Back/Front Motor Torque [Nm Nm]) -> [SecondaryBackFrontTorque]
  Secondary Leg Behavior/2(Secondary Force or Position Control [1/0]) -> [SecondaryForcePositionControl]
  Mux21/1 -> [TorsoYaw]
  Mux23/1 -> [TorsoRoll]
  Mux7/1 -> [TorsoPitch]
  [dqRoll] -> Mux23/2
  [dqPitch] -> Mux7/2
  [qLatR] -> lateral_coordinates/1
  [dqLatR] -> Gain12/1
  [qLatL] -> lateral_coordinates1/1
  [dqLatL] -> Gain13/1
  Mux22/1 -> [RLegRoll]
  Mux24/1 -> [LLegRoll]
  lateral_coordinates/1 -> Mux22/1
  lateral_coordinates1/1 -> Mux24/1
  Gain13/1 -> Mux24/2
  Gain12/1 -> Mux22/2
  Selector8/1 -> [dqLatL]
  Selector11/1 -> [dqLatR]
  Selector12/1 -> [dqBackR]
  Selector13/1 -> [dqFrontR]
  Selector9/1 -> [dqBackL]
  Selector10/1 -> [dqFrontL]
  Selector20/1 -> [dqPitch]
  Selector22/1 -> [dqYaw]
  Selector21/1 -> [dqRoll]
  dq/1 -> Selector10/1, [dq], Selector11/1, Selector21/1, Selector20/1, Selector22/1, Selector8/1, Selector12/1, Selector13/1, Selector9/1
  [qRoll] -> Mux23/1
  [qPitch] -> Mux7/1
  [qYaw] -> Mux21/1
  [dqYaw] -> Mux21/2

== system vertical_smm_with_lqr_3d/Control/Filter Velocities ==
  raw dq : Inport
  Demux : Demux  Outputs=3
  Demux1 : Demux  Outputs=3
  Demux2 : Demux  Outputs=2
  Demux3 : Demux  Outputs=2
  Fourbar : Selector  InputPortWidth=13  Indices=[1 2 3 4 5 6 7 8]
  Fourbar Velocity Filter : Scope  NumInputPorts=4
      settings: YMin=-0.55~-0.4~-0.4~-0.6  YMax=0.25~0.7~0.45~0.5  SaveName=ScopeData14  SampleInput=on
  IMU Two Pole Filter : DiscreteTransferFcn  Numerator=[A_lpf_imu 0 0]  Denominator=[1 B1_lpf_imu B2_lpf_imu]  SampleTime=sample_time
  Lateral : Selector  InputPortWidth=13  Indices=[9 10]
  Lateral Angle Two Pole Filter1 : DiscreteTransferFcn  Numerator=[A_lpf_lateral_angle 0 0]  Denominator=[1 B1_lpf_lateral_angle B2_lpf_lateral_angle]  SampleTime=sample_time
  Lateral Angle Two Pole Filter2 : DiscreteTransferFcn  Numerator=[A_lpf_fourbar_angles 0 0]  Denominator=[1 B1_lpf_fourbar_angles B2_lpf_fourbar_angles]  SampleTime=sample_time
  Leg Roll Velocity Filter : Scope  NumInputPorts=2
      settings: YMin=-0.225~-1.5  YMax=0.175~2.25  SaveName=LegRollFilter  SampleInput=on
  Mux : Mux  Inputs=3
  Mux{25..33} (9 alike) : Mux  Inputs=2
  Selector1 : Selector  InputPortWidth=8  Indices=[1 2]
  Selector2 : Selector  InputPortWidth=8  Indices=[3 4]
  Selector3 : Selector  InputPortWidth=8  Indices=[5 6]
  Selector34 : Selector  InputPortWidth=8  Indices=[1 2]
  Selector35 : Selector  InputPortWidth=8  Indices=[3 4]
  Selector36 : Selector  InputPortWidth=8  Indices=[5 6]
  Selector37 : Selector  InputPortWidth=8  Indices=[7 8]
  Selector4 : Selector  InputPortWidth=8  Indices=[7 8]
  Torso Orientation : Selector  InputPortWidth=13  Indices=[11 12 13]
  Torso Orientation Filter : Scope  NumInputPorts=3
      settings: YMin=-0.2~-0.03~-0.15  YMax=0.125~0.0275~0.15  SaveName=ScopeData13  SampleInput=on
  filtered dq : Outport
  wires:
  Lateral Angle Two Pole Filter2/1 -> Selector4/1, Selector3/1, Selector2/1, Selector1/1, Mux/1
  IMU Two Pole Filter/1 -> Demux1/1, Mux/3
  Mux/1 -> filtered dq/1
  raw dq/1 -> Fourbar/1, Torso Orientation/1, Lateral/1
  Lateral/1 -> Demux2/1, Lateral Angle Two Pole Filter1/1
  Torso Orientation/1 -> IMU Two Pole Filter/1, Demux/1
  Lateral Angle Two Pole Filter1/1 -> Demux3/1, Mux/2
  Mux25/1 -> Torso Orientation Filter/1
  Mux27/1 -> Torso Orientation Filter/3
  Mux26/1 -> Torso Orientation Filter/2
  Mux30/1 -> Fourbar Velocity Filter/1
  Mux32/1 -> Fourbar Velocity Filter/3
  Mux31/1 -> Fourbar Velocity Filter/2
  Mux33/1 -> Fourbar Velocity Filter/4
  Selector34/1 -> Mux30/1
  Fourbar/1 -> Selector34/1, Selector35/1, Selector36/1, Selector37/1, Lateral Angle Two Pole Filter2/1
  Selector35/1 -> Mux31/1
  Selector36/1 -> Mux32/1
  Selector37/1 -> Mux33/1
  Mux28/1 -> Leg Roll Velocity Filter/1
  Mux29/1 -> Leg Roll Velocity Filter/2
  Demux/1 -> Mux25/1
  Demux/2 -> Mux26/1
  Demux/3 -> Mux27/1
  Demux1/1 -> Mux25/2
  Demux1/2 -> Mux26/2
  Demux1/3 -> Mux27/2
  Demux2/2 -> Mux29/1
  Demux2/1 -> Mux28/1
  Demux3/1 -> Mux28/2
  Demux3/2 -> Mux29/2
  Selector4/1 -> Mux33/2
  Selector3/1 -> Mux32/2
  Selector2/1 -> Mux31/2
  Selector1/1 -> Mux30/2

== system vertical_smm_with_lqr_3d/Fourbar Gearside Kalman Filter/Pitch Offset ==
  in : Inport
  Constant2 : Constant  Value=torso_centerline_pitch_offset_angle
  Sum : Sum  Inputs=++|
  out : Outport
  wires:
  Constant2/1 -> Sum/1
  Sum/1 -> out/1
  in/1 -> Sum/2

== system vertical_smm_with_lqr_3d/Control/Behavior Control/Begin Hopping ==
  Enable : EnablePort  StatesWhenEnabling=reset
  Constant : Constant
  Hopping? : Outport  InitialOutput=[0]
  wires:
  Constant/1 -> Hopping?/1

== system vertical_smm_with_lqr_3d/Control/Behavior Control/Contact State Machine ==
  Contact Factor [body weight] : Inport
  "[Z dZ] [m m/s]" : Inport  Port=2
  Detect Fall Nonpositive : simulink/Logic and Bit Operations/Detect Fall Nonpositive  vinit=0  InputProcessing=Inherited  OutDataTypeStr=boolean
  Mux25 : Mux  Inputs=5
  Selector : Selector  InputPortWidth=2  Indices=[2]
  State Machine : State Transition Table  TreatAsAtomicUnit=on
  Terminator8 : Terminator
  Unit Delay5 : UnitDelay  SampleTime=-1
  Unit Delay6 : UnitDelay  SampleTime=sample_time
  Unit Delay7 : UnitDelay  SampleTime=sample_time
  Unit Delay8 : UnitDelay  SampleTime=sample_time
  flight [1/0] : Outport
  Exiting Stance [1/0] : Outport  Port=2
  wires:
  Detect Fall Nonpositive/1 -> Exiting Stance [1/0]/1
  Unit Delay7/1 -> flight [1/0]/1
  Unit Delay6/1 -> Detect Fall Nonpositive/1
  State Machine/4(" Takeoff") -> Unit Delay6/1, Mux25/4
  Unit Delay8/1 -> Terminator8/1
  Selector/1 -> State Machine/1(z_velocity), Unit Delay5/1
  Contact Factor [body weight]/1 -> State Machine/3(vertical_grf)
  Unit Delay5/1 -> State Machine/2(previous_z_velocity)
  State Machine/5(" Flight") -> Mux25/5, Unit Delay7/1
  Mux25/1 -> Unit Delay8/1
  State Machine/3(" Unloading") -> Mux25/3
  State Machine/2(" LockedContact") -> Mux25/2
  State Machine/1(" TouchDown") -> Mux25/1
  "[Z dZ] [m m/s]"/1 -> Selector/1

== system vertical_smm_with_lqr_3d/Control/Behavior Control/Desired Torque Derivative ==
  x : Inport
  flight [1/0] : Inport  Port=2
  Detect Change : simulink/Logic and Bit Operations/Detect Change  vinit=0  InputProcessing=Inherited  OutDataTypeStr=boolean
  Gain1 : Gain  Gain=1/sample_time
  Logical Operator : Logic  Operator=NOT  AllPortsSameDT=off  OutDataTypeStr=boolean
  Product : Product
  difference : simulink/Discrete/Difference  ICPrevInput=0.0  InputProcessing=Inherited  OutMin=[]  OutMax=[]  OutDataType=fixdt(1, 16)  OutScaling=2^-10  DoSatur=off
  two_pole_filter : DiscreteTransferFcn  Numerator=[A_lpf_dtau 0 0]  Denominator=[1 B1_lpf_dtau B2_lpf_dtau]  ExternalReset=Either  SampleTime=sample_time
      settings: InputPortMap=u0,r7
  dx/dt : Outport
  wires:
  Logical Operator/1 -> Product/2
  Detect Change/1 -> Logical Operator/1
  Product/1 -> two_pole_filter/1
  difference/1 -> Product/1
  flight [1/0]/1 -> Detect Change/1, two_pole_filter/2
  two_pole_filter/1 -> dx/dt/1
  x/1 -> Gain1/1
  Gain1/1 -> difference/1

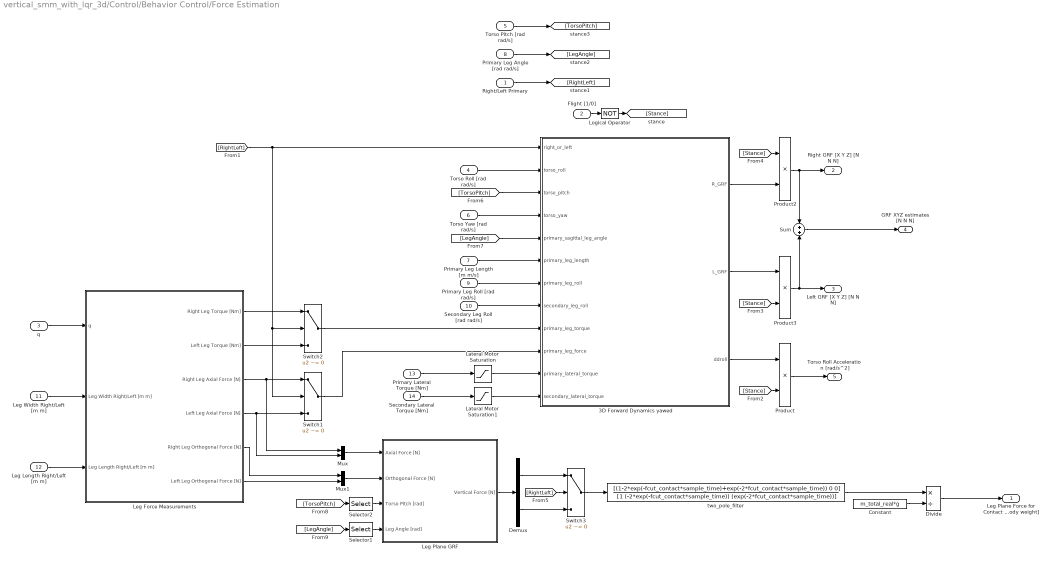
== system vertical_smm_with_lqr_3d/Control/Behavior Control/Force Estimation ==
  Right/Left Primary : Inport
  Flight [1/0] : Inport  Port=2
  q : Inport  Port=3
  Torso Roll [rad rad/s] : Inport  Port=4
  Torso Pitch [rad rad/s] : Inport  Port=5
  Torso Yaw [rad rad/s] : Inport  Port=6
  Primary Leg Length [m m/s] : Inport  Port=7
  Primary Leg Angle [rad rad/s] : Inport  Port=8
  Primary Leg Roll [rad rad/s] : Inport  Port=9
  Secondary Leg Roll [rad rad/s] : Inport  Port=10
  Leg Width Right/Left [m m] : Inport  Port=11
  Leg Length Right/Left [m m] : Inport  Port=12
  Primary Lateral Torque [Nm] : Inport  Port=13
  Secondary Lateral Torque [Nm] : Inport  Port=14
  3D Forward Dynamics yawed : MATLAB Function  TreatAsAtomicUnit=on
  Constant : Constant  Value=m_total_real*g
  Demux : Demux  Outputs=2
  Divide : Product  Inputs=*/
  Lateral Motor Saturation : Saturate  UpperLimit=HIP_MTR_MAX_TORQUE  LowerLimit=-HIP_MTR_MAX_TORQUE
      settings: AttributesFormatString=Top: %<UpperLimit>\nBottom: %<LowerLimit>
  Lateral Motor Saturation1 : Saturate  UpperLimit=HIP_MTR_MAX_TORQUE  LowerLimit=-HIP_MTR_MAX_TORQUE
      settings: AttributesFormatString=Top: %<UpperLimit>\nBottom: %<LowerLimit>
  Leg Force Measurements : Subsystem
  Leg Plane GRF : Subsystem
  Logical Operator : Logic  Operator=NOT  AllPortsSameDT=off  OutDataTypeStr=boolean
  Mux : Mux  Inputs=2
  Mux1 : Mux  Inputs=2
  Product : Product
  Product2 : Product
  Product3 : Product
  Selector1 : Selector  InputPortWidth=2  Indices=[1]
  Selector2 : Selector  InputPortWidth=2  Indices=[1]
  Sum : Sum  Inputs=+|+
  Switch1 : Switch  Criteria=u2 ~= 0
  Switch2 : Switch  Criteria=u2 ~= 0
  Switch3 : Switch  Criteria=u2 ~= 0
  two_pole_filter : DiscreteTransferFcn  Numerator=[(1-2*exp(-fcut_contact*sample_time)+exp(-2*fcut_contact*sample_time)) 0 0]  Denominator=[1 (-2*exp(-fcut_contact*sample_time)) (exp(-2*fcut_contact*sample_time))]  SampleTime=sample_time
  Leg Plane Force for Contact Detection [body weight] : Outport
  Right GRF [X Y Z] [N N N] : Outport  Port=2
  Left GRF [X Y Z] [N N N] : Outport  Port=3
  GRF XYZ estimates [N N N] : Outport  Port=4  OutputWhenDisabled=reset  InitialOutput=[0 0 0 0 0 0]
  Torso Roll Acceleration [rad/s^2] : Outport  Port=5  OutputWhenDisabled=reset  InitialOutput=[0 0 0 0 0 0]
  wires:
  Divide/1 -> Leg Plane Force for Contact Detection [body weight]/1
  Leg Width Right/Left [m m]/1 -> Leg Force Measurements/2(Leg Width Right/Left [m m])
  q/1 -> Leg Force Measurements/1(q)
  two_pole_filter/1 -> Divide/1
  Constant/1 -> Divide/2
  [RightLeft] -> 3D Forward Dynamics yawed/1(right_or_left), Switch2/2, Switch1/2
  Leg Length Right/Left [m m]/1 -> Leg Force Measurements/3(Leg Length Right/Left [m m])
  3D Forward Dynamics yawed/1(R_GRF) -> Product2/2
  3D Forward Dynamics yawed/2(L_GRF) -> Product3/1
  3D Forward Dynamics yawed/3(ddroll) -> Product/1
  Leg Force Measurements/3(Right Leg Axial Force [N]) -> Mux/1, Switch1/1
  Leg Force Measurements/4(Left Leg Axial Force [N]) -> Switch1/3, Mux/2
  Switch1/1 -> 3D Forward Dynamics yawed/10(primary_leg_force)
  [TorsoPitch] -> 3D Forward Dynamics yawed/3(torso_pitch)
  Torso Roll [rad rad/s]/1 -> 3D Forward Dynamics yawed/2(torso_roll)
  Torso Yaw [rad rad/s]/1 -> 3D Forward Dynamics yawed/4(torso_yaw)
  Primary Leg Length [m m/s]/1 -> 3D Forward Dynamics yawed/6(primary_leg_length)
  [LegAngle] -> 3D Forward Dynamics yawed/5(primary_sagittal_leg_angle)
  Flight [1/0]/1 -> Logical Operator/1
  [Stance] -> Product/2
  Product/1 -> Torso Roll Acceleration [rad/s^2]/1
  Switch3/1 -> two_pole_filter/1
  Logical Operator/1 -> [Stance]
  Product3/1 -> Left GRF [X Y Z] [N N N]/1, Sum/2
  Product2/1 -> Right GRF [X Y Z] [N N N]/1, Sum/1
  [Stance] -> Product3/2
  [Stance] -> Product2/1
  Primary Leg Roll [rad rad/s]/1 -> 3D Forward Dynamics yawed/7(primary_leg_roll)
  Secondary Leg Roll [rad rad/s]/1 -> 3D Forward Dynamics yawed/8(secondary_leg_roll)
  Switch2/1 -> 3D Forward Dynamics yawed/9(primary_leg_torque)
  Leg Force Measurements/1(Right Leg Torque [Nm]) -> Switch2/1
  Leg Force Measurements/2(Left Leg Torque [Nm]) -> Switch2/3
  Sum/1 -> GRF XYZ estimates [N N N]/1
  Mux1/1 -> Leg Plane GRF/2(Orthogonal Force [N])
  Mux/1 -> Leg Plane GRF/1(Axial Force [N])
  Leg Force Measurements/5(Right Leg Orthogonal Force [N]) -> Mux1/1
  Leg Force Measurements/6(Left Leg Orthogonal Force [N]) -> Mux1/2
  Right/Left Primary/1 -> [RightLeft]
  [RightLeft] -> Switch3/2
  Leg Plane GRF/1(Vertical Force [N]) -> Demux/1
  Demux/1 -> Switch3/1
  Demux/2 -> Switch3/3
  Primary Leg Angle [rad rad/s]/1 -> [LegAngle]
  Torso Pitch [rad rad/s]/1 -> [TorsoPitch]
  [LegAngle] -> Selector1/1
  Selector1/1 -> Leg Plane GRF/4(Leg Angle [rad])
  [TorsoPitch] -> Selector2/1
  Selector2/1 -> Leg Plane GRF/3(Torso Pitch [rad])
  Primary Lateral Torque [Nm]/1 -> Lateral Motor Saturation/1
  Secondary Lateral Torque [Nm]/1 -> Lateral Motor Saturation1/1
  Lateral Motor Saturation/1 -> 3D Forward Dynamics yawed/11(primary_lateral_torque)
  Lateral Motor Saturation1/1 -> 3D Forward Dynamics yawed/12(secondary_lateral_torque)

== system vertical_smm_with_lqr_3d/Control/Behavior Control/L Leg Calculator ==
  Front [rad rad/s] : Inport
  Back [rad rad/s] : Inport  Port=2
  Constant : Constant  Value=d_ankle_to_foot-0.01
  Demux1 : Demux  Outputs=2
  Gain1 : Gain  Gain=2*l_seg
  Gain2 : Gain  Gain=l_seg
  Gain3 : Gain  Gain=-1
  Gain4 : Gain  Gain=0.5
  Gain5 : Gain  Gain=0.5
  Gain6 : Gain  Gain=2
  Mux1 : Mux  Inputs=2
  Product : Product  RndMeth=Zero
  Sum : Sum  Inputs=++|
  Sum4 : Sum  Inputs=+|+
  Sum5 : Sum  Inputs=+|-
  Trigonometric Function : Trigonometry  Operator=cos
  Trigonometric Function1 : Trigonometry
  "Leg Length [m m/s] " : Outport
  Leg Angle [rad rad/s] : Outport  Port=2
  Leg Splay [rad rad/s] : Outport  Port=3
  w [m] : Outport  Port=4
  wires:
  Sum/1 -> Mux1/1
  Constant/1 -> Sum/1
  Sum4/1 -> Gain5/1
  Mux1/1 -> "Leg Length [m m/s] "/1
  Sum5/1 -> Demux1/1, Leg Splay [rad rad/s]/1
  Gain2/1 -> Gain6/1, Product/1
  Demux1/1 -> Gain4/1
  Gain3/1 -> Product/2
  Demux1/2 -> Gain3/1
  Back [rad rad/s]/1 -> Sum5/1, Sum4/1
  Front [rad rad/s]/1 -> Sum4/2, Sum5/2
  Product/1 -> Mux1/2
  Trigonometric Function1/1 -> Gain2/1
  Gain1/1 -> Sum/2
  Trigonometric Function/1 -> Gain1/1
  Gain4/1 -> Trigonometric Function/1, Trigonometric Function1/1
  Gain6/1 -> w [m]/1
  Gain5/1 -> Leg Angle [rad rad/s]/1
